simulink model "Gyro_sim"  (R2016b)
settings: Solver=ode4  StartTime=0.0  StopTime=inf  FixedStep=0.001  RelTol=1e-3
undefined symbols (not defined in the file or in its folder): serial
libraries: instrumentlib x2
settings Model: Creator=lenovo  LastModifiedBy=lenovo

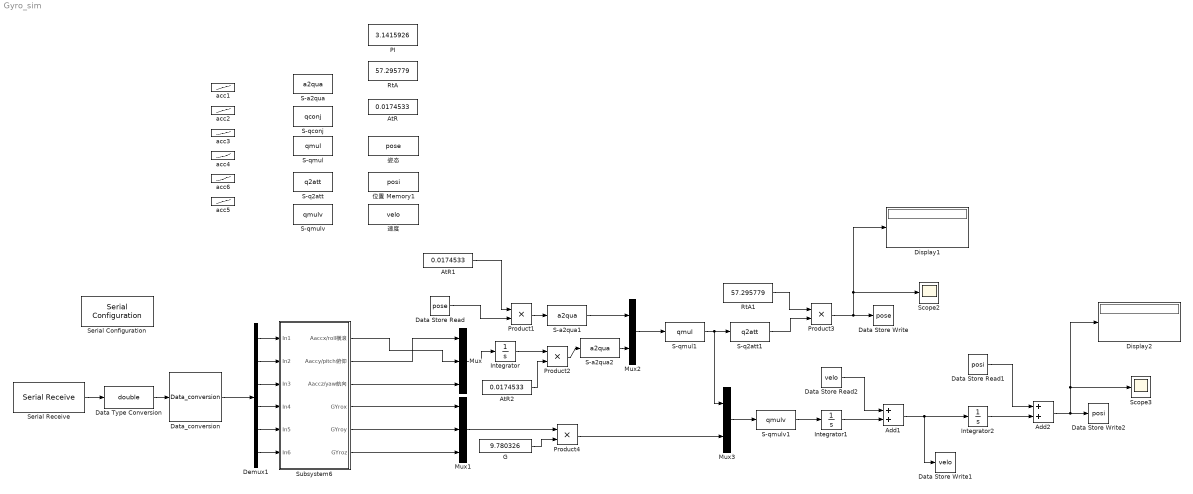
== system Gyro_sim ==
  Add1 : Sum
  Add2 : Sum
  AtR : Constant  Value=0.0174533
  AtR1 : Constant  Value=0.0174533
  AtR2 : Constant  Value=0.0174533
  Data Store Read : DataStoreRead  DataStoreName=pose
  Data Store Read1 : DataStoreRead  DataStoreName=posi
  Data Store Read2 : DataStoreRead  DataStoreName=velo
  Data Store Write : DataStoreWrite  DataStoreName=pose
  Data Store Write1 : DataStoreWrite  DataStoreName=velo
  Data Store Write2 : DataStoreWrite  DataStoreName=posi
  Data Type Conversion : DataTypeConversion  OutDataTypeStr=double
  Data_conversion : S-Function  FunctionName=Data_conversion  SFunctionDeploymentMode=off  EnableBusSupport=off
  Demux1 : Demux  Outputs=6
  Display1 : Display
  Display2 : Display
  G : Constant  Value=9.780326
  Integrator : Integrator
  Integrator1 : Integrator
  Integrator2 : Integrator
  Mux : Mux  Inputs=3
  Mux1 : Mux  Inputs=3
  Mux2 : Mux  Inputs=2
  Mux3 : Mux  Inputs=2
  PI : Constant  Value=3.1415926
  Product{1..4} (4 alike) : Product
  RtA : Constant  Value=57.295779
  RtA1 : Constant  Value=57.295779
  S-a2qua : S-Function  FunctionName=a2qua  SFunctionDeploymentMode=off  EnableBusSupport=off
  S-a2qua1 : S-Function  FunctionName=a2qua  SFunctionDeploymentMode=off  EnableBusSupport=off
  S-a2qua2 : S-Function  FunctionName=a2qua  SFunctionDeploymentMode=off  EnableBusSupport=off
  S-q2att : S-Function  FunctionName=q2att  SFunctionDeploymentMode=off  EnableBusSupport=off
  S-q2att1 : S-Function  FunctionName=q2att  SFunctionDeploymentMode=off  EnableBusSupport=off
  S-qconj : S-Function  FunctionName=qconj  SFunctionDeploymentMode=off  EnableBusSupport=off
  S-qmul : S-Function  FunctionName=qmul  SFunctionDeploymentMode=off  EnableBusSupport=off
  S-qmul1 : S-Function  FunctionName=qmul  SFunctionDeploymentMode=off  EnableBusSupport=off
  S-qmulv : S-Function  FunctionName=qmulv  SFunctionDeploymentMode=off  EnableBusSupport=off
  S-qmulv1 : S-Function  FunctionName=qmulv  SFunctionDeploymentMode=off  EnableBusSupport=off
  Scope2 : Scope
  Scope3 : Scope
  Serial Configuration : instrumentlib/Serial Configuration  Priority=-200000  ComPortMenu=<Please select a port...>  ComPort=COM4  ObjConstructor=serial('COM4');  BaudRate=115200  DataBits=8  Parity=none  StopBits=1  FlowControl=none  Timeout=10  ByteOrder=LittleEndian
  Serial Receive : instrumentlib/Serial Receive  ComPortMenu=<Please select a port...>  ComPort=COM4  ObjConstructor=serial('COM4');  Terminator=<none>  DataSize="[1  29]"  DataType=uint8  EnableBlockingMode=on  ActionDataUnavailable=Output last received value  CustomValue=0  SampleTime=0.001
  Subsystem6 : Subsystem
  acc{1..6} (6 alike) : Lookup  InputValues=[-0.0185 1.005]  Table=[0 1]  SaturateOnIntegerOverflow=on
  位置 Memory1 : DataStoreMemory  DataStoreName=posi  ReadBeforeWriteMsg=warning  WriteAfterWriteMsg=warning  WriteAfterReadMsg=warning  InitialValue=[0,0,0]  ShowAdditionalParam=off  OutDataTypeStr=double
  "姿态 " : DataStoreMemory  DataStoreName=pose  ReadBeforeWriteMsg=warning  WriteAfterWriteMsg=warning  WriteAfterReadMsg=warning  InitialValue=[0,0,0]  ShowAdditionalParam=off  OutDataTypeStr=double
  速度 : DataStoreMemory  DataStoreName=velo  ReadBeforeWriteMsg=warning  WriteAfterWriteMsg=warning  WriteAfterReadMsg=warning  InitialValue=[0,0,0]  ShowAdditionalParam=off  OutDataTypeStr=double
  wires:
  Data Type Conversion/1 -> Data_conversion/1
  Serial Receive/1 -> Data Type Conversion/1
  Data_conversion/1 -> Demux1/1
  Demux1/2 -> Subsystem6/2(In2)
  Demux1/1 -> Subsystem6/1(In1)
  Demux1/3 -> Subsystem6/3(In3)
  Demux1/4 -> Subsystem6/4(In4)
  Demux1/5 -> Subsystem6/5(In5)
  Demux1/6 -> Subsystem6/6(In6)
  Subsystem6/2(Aaccy/pitch俯仰) -> Mux/1
  Subsystem6/1(Aaccx/roll横滚) -> Mux/2
  Subsystem6/3(Aaccz/yaw航向) -> Mux/3
  Data Store Read/1 -> Product1/2
  Mux/1 -> Integrator/1
  S-a2qua1/1 -> Mux2/1
  Mux2/1 -> S-qmul1/1
  S-qmul1/1 -> Mux3/1, S-q2att1/1
  S-a2qua2/1 -> Mux2/2
  AtR1/1 -> Product1/1
  AtR2/1 -> Product2/2
  Product1/1 -> S-a2qua1/1
  Integrator/1 -> Product2/1
  Product2/1 -> S-a2qua2/1
  RtA1/1 -> Product3/1
  S-q2att1/1 -> Product3/2
  Product3/1 -> Scope2/1, Display1/1, Data Store Write/1
  Subsystem6/4(GYrox) -> Mux1/1
  Subsystem6/5(GYroy) -> Mux1/2
  Subsystem6/6(GYroz) -> Mux1/3
  Mux1/1 -> Product4/1
  G/1 -> Product4/2
  Product4/1 -> Mux3/2
  Mux3/1 -> S-qmulv1/1
  S-qmulv1/1 -> Integrator1/1
  Data Store Read2/1 -> Add1/1
  Integrator1/1 -> Add1/2
  Add1/1 -> Data Store Write1/1, Integrator2/1
  Integrator2/1 -> Add2/2
  Data Store Read1/1 -> Add2/1
  Add2/1 -> Display2/1, Scope3/1, Data Store Write2/1

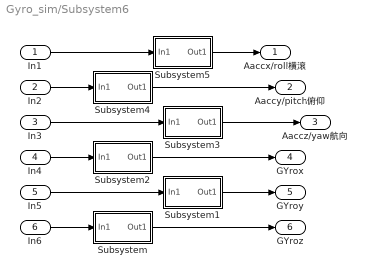
== system Gyro_sim/Subsystem6 ==
  In1 : Inport
  In2 : Inport  Port=2
  In3 : Inport  Port=3
  In4 : Inport  Port=4
  In5 : Inport  Port=5
  In6 : Inport  Port=6
  Subsystem : Subsystem
  Subsystem1 : Subsystem
  Subsystem2 : Subsystem
  Subsystem3 : Subsystem
  Subsystem4 : Subsystem
  Subsystem5 : Subsystem
  Aaccx/roll横滚 : Outport
  Aaccy/pitch俯仰 : Outport  Port=2
  Aaccz/yaw航向 : Outport  Port=3
  GYrox : Outport  Port=4
  GYroy : Outport  Port=5
  GYroz : Outport  Port=6
  wires:
  In1/1 -> Subsystem5/1(In1)
  In3/1 -> Subsystem3/1(In1)
  In2/1 -> Subsystem4/1(In1)
  In5/1 -> Subsystem1/1(In1)
  In6/1 -> Subsystem/1(In1)
  Subsystem/1(Out1) -> GYroz/1
  Subsystem1/1(Out1) -> GYroy/1
  In4/1 -> Subsystem2/1(In1)
  Subsystem3/1(Out1) -> Aaccz/yaw航向/1
  Subsystem4/1(Out1) -> Aaccy/pitch俯仰/1
  Subsystem5/1(Out1) -> Aaccx/roll横滚/1
  Subsystem2/1(Out1) -> GYrox/1

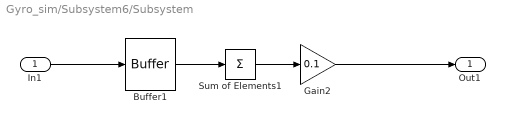
== system Gyro_sim/Subsystem6/Subsystem ==
  In1 : Inport
  Buffer1 : Buffer  N=10  V=9  TreatMby1Signals=One channel  OutputFrames=off
  Gain2 : Gain  Gain=0.1
  Sum of Elements1 : Sum  Inputs=+
  Out1 : Outport
  wires:
  Buffer1/1 -> Sum of Elements1/1
  Sum of Elements1/1 -> Gain2/1
  In1/1 -> Buffer1/1
  Gain2/1 -> Out1/1

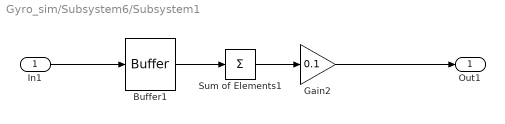
== system Gyro_sim/Subsystem6/Subsystem1 ==
  In1 : Inport
  Buffer1 : Buffer  N=10  V=9  TreatMby1Signals=One channel  OutputFrames=off
  Gain2 : Gain  Gain=0.1
  Sum of Elements1 : Sum  Inputs=+
  Out1 : Outport
  wires:
  Gain2/1 -> Out1/1
  In1/1 -> Buffer1/1
  Sum of Elements1/1 -> Gain2/1
  Buffer1/1 -> Sum of Elements1/1

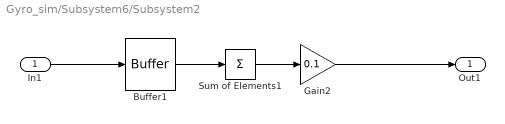
== system Gyro_sim/Subsystem6/Subsystem2 ==
  In1 : Inport
  Buffer1 : Buffer  N=10  V=9  TreatMby1Signals=One channel  OutputFrames=off
  Gain2 : Gain  Gain=0.1
  Sum of Elements1 : Sum  Inputs=+
  Out1 : Outport
  wires:
  Buffer1/1 -> Sum of Elements1/1
  Sum of Elements1/1 -> Gain2/1
  In1/1 -> Buffer1/1
  Gain2/1 -> Out1/1

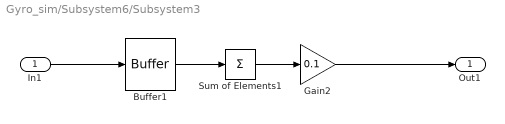
== system Gyro_sim/Subsystem6/Subsystem3 ==
  In1 : Inport
  Buffer1 : Buffer  N=10  V=9  TreatMby1Signals=One channel  OutputFrames=off
  Gain2 : Gain  Gain=0.1
  Sum of Elements1 : Sum  Inputs=+
  Out1 : Outport
  wires:
  Gain2/1 -> Out1/1
  In1/1 -> Buffer1/1
  Sum of Elements1/1 -> Gain2/1
  Buffer1/1 -> Sum of Elements1/1

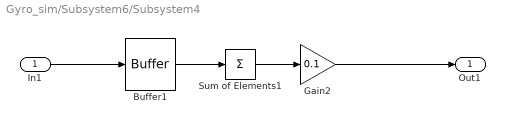
== system Gyro_sim/Subsystem6/Subsystem4 ==
  In1 : Inport
  Buffer1 : Buffer  N=10  V=9  TreatMby1Signals=One channel  OutputFrames=off
  Gain2 : Gain  Gain=0.1
  Sum of Elements1 : Sum  Inputs=+
  Out1 : Outport
  wires:
  Buffer1/1 -> Sum of Elements1/1
  Sum of Elements1/1 -> Gain2/1
  In1/1 -> Buffer1/1
  Gain2/1 -> Out1/1

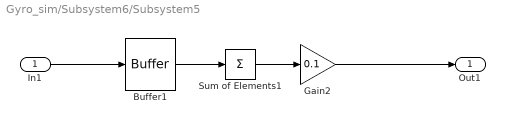
== system Gyro_sim/Subsystem6/Subsystem5 ==
  In1 : Inport
  Buffer1 : Buffer  N=10  V=9  TreatMby1Signals=One channel  OutputFrames=off
  Gain2 : Gain  Gain=0.1
  Sum of Elements1 : Sum  Inputs=+
  Out1 : Outport
  wires:
  Gain2/1 -> Out1/1
  In1/1 -> Buffer1/1
  Sum of Elements1/1 -> Gain2/1
  Buffer1/1 -> Sum of Elements1/1
